simulink model "GolfSwing3D_KineticallyDriven"  (R2025a)
settings: Solver=VariableStepAuto  StartTime=0.0  StopTime=StopTime  MaxStep=0.001  RelTol=1e-3
model workspace: external: MAT-File 3DModelInputs.mat (data not in the file)
undefined symbols (not defined in the file or in its folder): GripStrength, KillswitchFinalValue, KillswitchInitialValue, KillswitchStepTime, LeftLowerArmLength, PlaneTilt, RightLowerArmLength, UpperTorsoLength, X, Y, Z
libraries: nesl_utility x408, sm_lib x139, matrix_library x11, simulink x1
(part 11 of 14)

== matlab function GolfSwing3D_KineticallyDriven/Hip Input Function/Hip Torque Output ==
  data: JointTorqueHipX output; Time input; Killswitch input; HipPositionX input; HipPositionY input; HipPositionZ input; HipVelocityX input; HipVelocityY input; HipVelocityZ input; HipInputXA parameter; HipInputYA parameter; HipInputZA parameter; HipInputXB parameter; HipInputYB parameter; HipInputZB parameter; HipPositionSetpointX parameter; HipPositionSetpointY parameter; GlobalGain parameter; JointTorqueHipY output; JointTorqueHipZ output; HipDampeningX parameter; HipDampeningY parameter; HipDampeningZ parameter; HipConstantX parameter; HipConstantY parameter; HipConstantZ parameter; HipTimeGainX parameter; HipTimeGainY parameter; HipTimeGainZ parameter; HipInputZC parameter; HipInputXC parameter; HipInputYC parameter; HipPositionGainX parameter; HipPositionGainY parameter; HipPositionGainZ parameter; HipPositionSetpointZ parameter; TargetHipPositionX parameter; TargetHipPositionY parameter; TargetHipPositionZ parameter; TargetHipVelocityX parameter; TargetHipVelocityY parameter; TargetHipVelocityZ parameter; HipPCGainX parameter; HipPCGainY parameter; HipPCGainZ parameter; HipVCGainX parameter; HipVCGainY parameter; HipVCGainZ parameter; ModelingMode parameter; ZVCFHipTorqueX parameter; ZVCFHipTorqueY parameter; ZVCFHipTorqueZ parameter; GlobalPCGain parameter; GlobalVCGain parameter; DampeningGlobalGain parameter; TargetImpactTime parameter; HipPositionInputX output; HipPositionInputY output; HipPositionInputZ output; HipVelocityInputX output; HipVelocityInputY output; HipVelocityInputZ output; HipAccelerationInputX output; HipAccelerationInputY output; HipAccelerationInputZ output; HipStartPositionX parameter; HipStartPositionY parameter; HipStartPositionZ parameter; HipStartVelocityX parameter; HipStartVelocityY parameter; HipStartVelocityZ parameter; KinematicMode parameter; HipAoX parameter; HipAoY parameter; HipAoZ parameter; HipAfX parameter; HipAfY parameter; HipAfZ parameter; HipInputXD parameter; HipInputYD parameter; HipInputXE parameter; HipInputXF parameter; HipInputXG parameter; HipInputYE parameter; HipInputYF parameter; HipInputYG parameter; HipInputZD parameter; HipInputZE parameter; HipInputZF parameter; HipInputZG parameter
function [JointTorqueHipX,JointTorqueHipY,JointTorqueHipZ,HipPositionInputX,HipPositionInputY,HipPositionInputZ,HipVelocityInputX,...
    HipVelocityInputY, HipVelocityInputZ,HipAccelerationInputX,HipAccelerationInputY,HipAccelerationInputZ] = fcn(Time,Killswitch, HipPositionX,HipPositionY,HipPositionZ, HipVelocityX,HipVelocityY,...
    HipVelocityZ,...
    HipInputXA,HipInputYA,HipInputZA, HipInputXB,HipInputYB,HipInputZB, HipPositionSetpointX,HipPositionSetpointY,GlobalGain,...
    HipDampeningX, HipDampeningY, HipDampeningZ, HipConstantX, HipConstantY, HipConstantZ, HipTimeGainX, HipTimeGainY, HipTimeGainZ, HipInputZC,...
    HipInputXC, HipInputYC, HipPositionGainX, HipPositionGainY, HipPositionGainZ, HipPositionSetpointZ,...
    TargetHipPositionX, TargetHipPositionY, TargetHipPositionZ, TargetHipVelocityX, TargetHipVelocityY, TargetHipVelocityZ,HipPCGainX, HipPCGainY, HipPCGainZ, HipVCGainX,...
    HipVCGainY, HipVCGainZ,ModelingMode,ZVCFHipTorqueX, ZVCFHipTorqueY, ZVCFHipTorqueZ,GlobalPCGain, GlobalVCGain,DampeningGlobalGain,TargetImpactTime,HipStartPositionX,...
    HipStartPositionY, HipStartPositionZ, HipStartVelocityX, HipStartVelocityY, HipStartVelocityZ,KinematicMode,HipAoX, HipAoY, HipAoZ,HipAfX, HipAfY, HipAfZ,...
    HipInputXD, HipInputYD, HipInputXE, HipInputXF, HipInputXG, HipInputYE, HipInputYF, HipInputYG, HipInputZD, HipInputZE, HipInputZF, HipInputZG)

%Tau=Time/TargetImpactTime;
t=Time;

% %%%%%%%%%%%%%%%%%%%%%%%%%%%%%%%%%%%%%%%%%%%
% % Kinetic Input Selection and Calculation
% %%%%%%%%%%%%%%%%%%%%%%%%%%%%%%%%%%%%%%%%%%%

if ModelingMode==0
    % Values are all set to zero.
    JointTorqueHipX=0;
    JointTorqueHipY=0;
    JointTorqueHipZ=0;
elseif ModelingMode==1
    % Control based strategy. Values are based on difference in value
    % between the current state and desired state.
    % Hip Joint Rotational Deltas
    DeltaHipPositionX=HipPositionX-TargetHipPositionX;
    DeltaHipPositionY=HipPositionY-TargetHipPositionY;
    DeltaHipPositionZ=HipPositionZ-TargetHipPositionZ;
    DeltaHipVelocityX=HipVelocityX-TargetHipVelocityX;
    DeltaHipVelocityY=HipVelocityY-TargetHipVelocityY;
    DeltaHipVelocityZ=HipVelocityZ-TargetHipVelocityZ;
    % Control Based Strategy
    JointTorqueHipX=DeltaHipPositionX*HipPCGainX*GlobalPCGain-DeltaHipVelocityX*HipVCGainX*GlobalVCGain-DampeningGlobalGain*HipDampeningX*HipVelocityX;
    JointTorqueHipY=DeltaHipPositionY*HipPCGainY*GlobalPCGain-DeltaHipVelocityY*HipVCGainY*GlobalVCGain-DampeningGlobalGain*HipDampeningY*HipVelocityY;
    JointTorqueHipZ=DeltaHipPositionZ*HipPCGainZ*GlobalPCGain-DeltaHipVelocityZ*HipVCGainZ*GlobalVCGain-DampeningGlobalGain*HipDampeningZ*HipVelocityZ;
elseif ModelingMode==2
    % Forward Dynamics Based Strategy. Values are computed based on a
    % polynomial and a combination of dampening and position gained
    % factors.
    JointTorqueHipX=Killswitch*GlobalGain*(HipConstantX+HipTimeGainX*Time-HipPositionGainX*(HipPositionX-HipPositionSetpointX)...
    -HipDampeningX*HipVelocityX);
    JointTorqueHipY=Killswitch*GlobalGain*(HipConstantY+HipTimeGainY*Time-HipPositionGainY*(HipPositionY-HipPositionSetpointY)...
    -HipDampeningY*HipVelocityY);
    JointTorqueHipZ=Killswitch*GlobalGain*(HipConstantZ+HipTimeGainZ*Time-HipPositionGainZ*(HipPositionZ-HipPositionSetpointZ)...
    -HipDampeningZ*HipVelocityZ);
elseif ModelingMode==3
    JointTorqueHipX=HexPolyInputFunction(HipInputXA,HipInputXB,HipInputXC,HipInputXD,HipInputXE,HipInputXF,HipInputXG,Time)*Killswitch;
    JointTorqueHipY=HexPolyInputFunction(HipInputYA,HipInputYB,HipInputYC,HipInputYD,HipInputYE,HipInputYF,HipInputYG,Time)*Killswitch;
    JointTorqueHipZ=HexPolyInputFunction(HipInputZA,HipInputZB,HipInputZC,HipInputZD,HipInputZE,HipInputZF,HipInputZG,Time)*Killswitch;
else
    %ZVCF Based Joint Torques. Values are pulled from model workspace and
    %held constant.
    JointTorqueHipX=ZVCFHipTorqueX;
    JointTorqueHipY=ZVCFHipTorqueY;
    JointTorqueHipZ=ZVCFHipTorqueZ;
end

% %%%%%%%%%%%%%%%%%%%%%%%%%%%%%%%%%%%%%%%%%%%
% % Kinematic Input Selection and Calculation
% %%%%%%%%%%%%%%%%%%%%%%%%%%%%%%%%%%%%%%%%%%%

if KinematicMode==0
    % All kinematic values set to zero.
    HipPositionInputX=0;
    HipPositionInputY=0;
    HipPositionInputZ=0;
    HipVelocityInputX=0;
    HipVelocityInputY=0;
    HipVelocityInputZ=0;
    HipAccelerationInputX=0;
    HipAccelerationInputY=0;
    HipAccelerationInputZ=0;
elseif KinematicMode==1
    % 1st Order Acceleration, 2nd Order Velocity, 3rd Order Position Solution
    PTX=TargetHipPositionX;       
    VTX=TargetHipVelocityX;
    PTY=TargetHipPositionY;
    VTY=TargetHipVelocityY;
    PTZ=TargetHipPositionZ;
    VTZ=TargetHipVelocityZ;
    % Define Starting Position and Velocity
    PIX=HipStartPositionX;
    VIX=HipStartVelocityX;
    PIY=HipStartPositionY;
    VIY=HipStartVelocityY;
    PIZ=HipStartPositionZ;
    VIZ=HipStartVelocityZ;
    AX=3*((VTX+VIX)*TargetImpactTime-2*(PTX-PIX))/TargetImpactTime^3;         % Constant in position equation
    BX=-2*((VTX+2*VIX)*TargetImpactTime-3*(PTX-PIX))/TargetImpactTime^2;         % Constant in position equation
    CX=VIX;         % Starting Velocity at Time Zero
    DX=PIX;         % Starting Position at Time Zero
    AY=3*((VTY+VIY)*TargetImpactTime-2*(PTY-PIY))/TargetImpactTime^3;         % Constant in position equation
    BY=-2*((VTY+2*VIY)*TargetImpactTime-3*(PTY-PIY))/TargetImpactTime^2;         % Constant in position equation
    CY=VIY;         % Starting Velocity at Time Zero
    DY=PIY;         % Starting Position at Time Zero
    AZ=3*((VTZ+VIZ)*TargetImpactTime-2*(PTZ-PIZ))/TargetImpactTime^3;         % Constant in position equation
    BZ=-2*((VTZ+2*VIZ)*TargetImpactTime-3*(PTZ-PIZ))/TargetImpactTime^2;         % Constant in position equation
    CZ=VIZ;         % Starting Velocity at Time Zero
    DZ=PIZ;         % Starting Position at Time Zero
    % Equation for position as a function of time
    HipPositionInputX=AX*Time^3/3+BX*Time^2/2+CX*Time+DX;
    HipPositionInputY=AY*Time^3/3+BY*Time^2/2+CY*Time+DY;
    HipPositionInputZ=AZ*Time^3/3+BZ*Time^2/2+CZ*Time+DZ;
    HipVelocityInputX=AX*Time^2+BX*Time+CX;
    HipVelocityInputY=AY*Time^2+BY*Time+CY;
    HipVelocityInputZ=AZ*Time^2+BZ*Time+CZ;
    HipAccelerationInputX=2*AX*Time+BX;
    HipAccelerationInputY=2*AY*Time+BY;
    HipAccelerationInputZ=2*AZ*Time+BZ;
elseif KinematicMode==2
    % 2nd Order Acceleration, 3rd Order Velocity, 4th Order Position Solution
    Tt=TargetImpactTime;
    t=Time;
    PoX=HipStartPositionX;
    PoY=HipStartPositionY;
    PoZ=HipStartPositionZ;
    VoX=HipStartVelocityX;
    VoY=HipStartVelocityY;
    VoZ=HipStartVelocityZ;
    PfX=TargetHipPositionX;
    PfY=TargetHipPositionY;
    PfZ=TargetHipPositionZ;
    VfX=TargetHipVelocityX;
    VfY=TargetHipVelocityY;
    VfZ=TargetHipVelocityZ;
    AoX=HipAoX;
    AoY=HipAoY;
    AoZ=HipAoZ;
    HipPositionInputX=PoX + VoX*t + (AoX*t^2)/2 - (t^3*(4*PoX - 4*PfX + Tt*VfX + 3*Tt*VoX + AoX*Tt^2))/Tt^3 + (t^4*(6*PoX - 6*PfX + 2*Tt*VfX + 4*Tt*VoX + AoX*Tt^2))/(2*Tt^4);
    HipPositionInputY=PoY + VoY*t + (AoY*t^2)/2 - (t^3*(4*PoY - 4*PfY + Tt*VfY + 3*Tt*VoY + AoY*Tt^2))/Tt^3 + (t^4*(6*PoY - 6*PfY + 2*Tt*VfY + 4*Tt*VoY + AoY*Tt^2))/(2*Tt^4);
    HipPositionInputZ=PoZ + VoZ*t + (AoZ*t^2)/2 - (t^3*(4*PoZ - 4*PfZ + Tt*VfZ + 3*Tt*VoZ + AoZ*Tt^2))/Tt^3 + (t^4*(6*PoZ - 6*PfZ + 2*Tt*VfZ + 4*Tt*VoZ + AoZ*Tt^2))/(2*Tt^4);
    HipVelocityInputX=VoX + AoX*t - (3*t^2*(4*PoX - 4*PfX + Tt*VfX + 3*Tt*VoX + AoX*Tt^2))/Tt^3 + (2*t^3*(6*PoX - 6*PfX + 2*Tt*VfX + 4*Tt*VoX + AoX*Tt^2))/Tt^4;
    HipVelocityInputY=VoY + AoY*t - (3*t^2*(4*PoY - 4*PfY + Tt*VfY + 3*Tt*VoY + AoY*Tt^2))/Tt^3 + (2*t^3*(6*PoY - 6*PfY + 2*Tt*VfY + 4*Tt*VoY + AoY*Tt^2))/Tt^4;
    HipVelocityInputZ=VoZ + AoZ*t - (3*t^2*(4*PoZ - 4*PfZ + Tt*VfZ + 3*Tt*VoZ + AoZ*Tt^2))/Tt^3 + (2*t^3*(6*PoZ - 6*PfZ + 2*Tt*VfZ + 4*Tt*VoZ + AoZ*Tt^2))/Tt^4;
    HipAccelerationInputX=AoX + (6*t^2*(6*PoX - 6*PfX + 2*Tt*VfX + 4*Tt*VoX + AoX*Tt^2))/Tt^4 - (6*t*(4*PoX - 4*PfX + Tt*VfX + 3*Tt*VoX + AoX*Tt^2))/Tt^3;
    HipAccelerationInputY=AoY + (6*t^2*(6*PoY - 6*PfY + 2*Tt*VfY + 4*Tt*VoY + AoY*Tt^2))/Tt^4 - (6*t*(4*PoY - 4*PfY + Tt*VfY + 3*Tt*VoY + AoY*Tt^2))/Tt^3;
    HipAccelerationInputZ=AoZ + (6*t^2*(6*PoZ - 6*PfZ + 2*Tt*VfZ + 4*Tt*VoZ + AoZ*Tt^2))/Tt^4 - (6*t*(4*PoZ - 4*PfZ + Tt*VfZ + 3*Tt*VoZ + AoZ*Tt^2))/Tt^3;
else
    % 3rd Order Acceleration, 4th Order Velocity, 5th Order Position Solution
    Tt=TargetImpactTime;
    t=Time;
    PoX=HipStartPositionX;
    PoY=HipStartPositionY;
    PoZ=HipStartPositionZ;
    VoX=HipStartVelocityX;
    VoY=HipStartVelocityY;
    VoZ=HipStartVelocityZ;
    PfX=TargetHipPositionX;
    PfY=TargetHipPositionY;
    PfZ=TargetHipPositionZ;
    VfX=TargetHipVelocityX;
    VfY=TargetHipVelocityY;
    VfZ=TargetHipVelocityZ;
    AoX=HipAoX;
    AoY=HipAoY;
    AoZ=HipAoZ;
    AfX=HipAfX;
    AfY=HipAfY;
    AfZ=HipAfZ;
    HipPositionInputX=PoX+VoX*t+(AoX*t^2)/2-(t^5*(12*PoX-12*PfX+6*Tt*VfX+6*Tt*VoX-AfX*Tt^2+AoX*Tt^2))/(2*Tt^5)-(t^3*(20*PoX-20*PfX+8*Tt*VfX+12*Tt*VoX-AfX*Tt^2+3*AoX*Tt^2))/(2*Tt^3)+(t^4*(30*PoX-30*PfX+14*Tt*VfX+16*Tt*VoX-2*AfX*Tt^2+3*AoX*Tt^2))/(2*Tt^4);
    HipPositionInputY=PoY+VoY*t+(AoY*t^2)/2-(t^5*(12*PoY-12*PfY+6*Tt*VfY+6*Tt*VoY-AfY*Tt^2+AoY*Tt^2))/(2*Tt^5)-(t^3*(20*PoY-20*PfY+8*Tt*VfY+12*Tt*VoY-AfY*Tt^2+3*AoY*Tt^2))/(2*Tt^3)+(t^4*(30*PoY-30*PfY+14*Tt*VfY+16*Tt*VoY-2*AfY*Tt^2+3*AoY*Tt^2))/(2*Tt^4);  
    HipPositionInputZ=PoZ+VoZ*t+(AoZ*t^2)/2-(t^5*(12*PoZ-12*PfZ+6*Tt*VfZ+6*Tt*VoZ-AfZ*Tt^2+AoZ*Tt^2))/(2*Tt^5)-(t^3*(20*PoZ-20*PfZ+8*Tt*VfZ+12*Tt*VoZ-AfZ*Tt^2+3*AoZ*Tt^2))/(2*Tt^3)+(t^4*(30*PoZ-30*PfZ+14*Tt*VfZ+16*Tt*VoZ-2*AfZ*Tt^2+3*AoZ*Tt^2))/(2*Tt^4);
    HipVelocityInputX=VoX+AoX*t-(5*t^4*(12*PoX-12*PfX+6*Tt*VfX+6*Tt*VoX-AfX*Tt^2+AoX*Tt^2))/(2*Tt^5)-(3*t^2*(20*PoX-20*PfX+8*Tt*VfX+12*Tt*VoX-AfX*Tt^2+3*AoX*Tt^2))/(2*Tt^3)+(2*t^3*(30*PoX-30*PfX+14*Tt*VfX+16*Tt*VoX-2*AfX*Tt^2+3*AoX*Tt^2))/Tt^4;
    HipVelocityInputY=VoY+AoY*t-(5*t^4*(12*PoY-12*PfY+6*Tt*VfY+6*Tt*VoY-AfY*Tt^2+AoY*Tt^2))/(2*Tt^5)-(3*t^2*(20*PoY-20*PfY+8*Tt*VfY+12*Tt*VoY-AfY*Tt^2+3*AoY*Tt^2))/(2*Tt^3)+(2*t^3*(30*PoY-30*PfY+14*Tt*VfY+16*Tt*VoY-2*AfY*Tt^2+3*AoY*Tt^2))/Tt^4;
    HipVelocityInputZ=VoZ+AoZ*t-(5*t^4*(12*PoZ-12*PfZ+6*Tt*VfZ+6*Tt*VoZ-AfZ*Tt^2+AoZ*Tt^2))/(2*Tt^5)-(3*t^2*(20*PoZ-20*PfZ+8*Tt*VfZ+12*Tt*VoZ-AfZ*Tt^2+3*AoZ*Tt^2))/(2*Tt^3)+(2*t^3*(30*PoZ-30*PfZ+14*Tt*VfZ+16*Tt*VoZ-2*AfZ*Tt^2+3*AoZ*Tt^2))/Tt^4;
    HipAccelerationInputX=AoX-(3*t*(20*PoX-20*PfX+8*Tt*VfX+12*Tt*VoX-AfX*Tt^2+3*AoX*Tt^2))/Tt^3-(10*t^3*(12*PoX-12*PfX+6*Tt*VfX+6*Tt*VoX-AfX*Tt^2+AoX*Tt^2))/Tt^5+(6*t^2*(30*PoX-30*PfX+14*Tt*VfX+16*Tt*VoX-2*AfX*Tt^2+3*AoX*Tt^2))/Tt^4;
    HipAccelerationInputY=AoY-(3*t*(20*PoY-20*PfY+8*Tt*VfY+12*Tt*VoY-AfY*Tt^2+3*AoY*Tt^2))/Tt^3-(10*t^3*(12*PoY-12*PfY+6*Tt*VfY+6*Tt*VoY-AfY*Tt^2+AoY*Tt^2))/Tt^5+(6*t^2*(30*PoY-30*PfY+14*Tt*VfY+16*Tt*VoY-2*AfY*Tt^2+3*AoY*Tt^2))/Tt^4;
    HipAccelerationInputZ=AoZ-(3*t*(20*PoZ-20*PfZ+8*Tt*VfZ+12*Tt*VoZ-AfZ*Tt^2+3*AoZ*Tt^2))/Tt^3-(10*t^3*(12*PoZ-12*PfZ+6*Tt*VfZ+6*Tt*VoZ-AfZ*Tt^2+AoZ*Tt^2))/Tt^5+(6*t^2*(30*PoZ-30*PfZ+14*Tt*VfZ+16*Tt*VoZ-2*AfZ*Tt^2+3*AoZ*Tt^2))/Tt^4;
end

% Calculate Higher Order Derivatives of the Position Outputs
HipJerkX=gradient(HipAccelerationInputX,t);
HipJerkY=gradient(HipAccelerationInputY,t);
HipJerkZ=gradient(HipAccelerationInputZ,t);
HipSnapX=gradient(HipJerkX,t);
HIpSnapY=gradient(HipJerkY,t);
HipSnapZ=gradient(HipJerkZ,t);
HipCrackleX=gradient(HipSnapX,t);
HipCrackleY=gradient(HIpSnapY,t);
HipCrackleZ=gradient(HipSnapZ,t);
HipPopX=gradient(HipCrackleX,t);
HipPopY=gradient(HipCrackleY,t);
HipPopZ=gradient(HipCrackleZ,t);

== matlab function GolfSwing3D_KineticallyDriven/Club Calculations/Subsystem/Total Wrist Forces and Torques Local ==
  data: LHTL input; RHTL input; LHTG input; RHTG input; LHFL input; RHFL input; LHFG input; RHFG input; HandPathVector input; MidpointVelocity input; TotalHandTorqueLocal output; TotalHandTorqueGlobal output; ClubTorqueMagnitude output; TotalHandForceLocal output; TotalHandForceGlobal output; ClubForceMagnitude output; HandForceYankLocal output; ForceAlongHandPath output; LinearPoweronClub output; LHAV input; RHAV input; LHonClubAngularPower output; RHonClubAngularPower output; LHMOF input; RHMOF input; SumofMomentsLHonClub output; SumofMomentsRHonClub output; LHVelocity input; RHVelocity input; LHandPathVector input; RHandPathVector input; LHonClubLinearPower output; RHonClubLinearPower output; LHForceAlongHandPath output; RHForceAlongHandPath output
function [TotalHandTorqueLocal,TotalHandTorqueGlobal,ClubTorqueMagnitude,TotalHandForceLocal,TotalHandForceGlobal,...
    ClubForceMagnitude,HandForceYankLocal,ForceAlongHandPath,LinearPoweronClub,...
    LHonClubAngularPower,RHonClubAngularPower,SumofMomentsLHonClub,SumofMomentsRHonClub,...
    LHonClubLinearPower,RHonClubLinearPower,LHForceAlongHandPath,RHForceAlongHandPath] = ...
    fcn(LHTL,RHTL,LHTG,RHTG,LHFL,RHFL,LHFG,RHFG,HandPathVector,MidpointVelocity,LHAV,RHAV,LHMOF,RHMOF,...
    LHVelocity,RHVelocity,LHandPathVector,RHandPathVector)

% Local Torques
TotalHandTorqueLocal = LHTL+RHTL;
ClubTorqueMagnitude=norm(TotalHandTorqueLocal);

% Local Forces
TotalHandForceLocal = LHFL+RHFL;
ClubForceMagnitude=norm(TotalHandForceLocal);
HandForceYankLocal=diff(TotalHandForceLocal);

% Global Torques
TotalHandTorqueGlobal=LHTG+RHTG;

% Global Forces
TotalHandForceGlobal=LHFG+RHFG;

% Force Along Hand Path
ForceAlongHandPath=dot(TotalHandForceGlobal,HandPathVector);
LHForceAlongHandPath=dot(LHFG,LHandPathVector);
RHForceAlongHandPath=dot(RHFG,RHandPathVector);

% Linear Power Applied to Club
LinearPoweronClub=dot(TotalHandForceGlobal,MidpointVelocity);
LHonClubLinearPower=dot(LHFG,LHVelocity);
RHonClubLinearPower=dot(RHFG,RHVelocity);

% Angular Power
LHonClubAngularPower=dot(LHTG,LHAV);
RHonClubAngularPower=dot(RHTG,RHAV);

% Sum of Moments
SumofMomentsLHonClub=LHMOF+LHTG;
SumofMomentsRHonClub=RHMOF+RHTG;

== matlab function GolfSwing3D_KineticallyDriven/Torso Input Function/Torso Input Torque ==
  data: Time input; Killswitch input; JointTorqueTorso output; TorsoInputB parameter; TorsoPositionSetpoint parameter; GlobalGain parameter; TorsoDampening parameter; ModelingMode parameter; GlobalPCGain parameter; GlobalVCGain parameter; DampeningGlobalGain parameter; TargetImpactTime parameter; KinematicMode parameter; TorsoAo parameter; TorsoStartPosition parameter; TorsoStartVelocity parameter; ZVCFTorsoTorque parameter; TorsoPCGain parameter; TorsoVCGain parameter; TargetTorsoVelocity parameter; TargetTorsoPosition parameter; TorsoPositionGain parameter; TorsoPositionInput output; TorsoVelocityInput output; TorsoAccelerationInput output; TorsoInputC parameter; TorsoTimeGain parameter; TorsoConstant parameter; TorsoPosition input; TorsoVelocity input; TorsoInputA parameter; TorsoAf parameter; TorsoInputD parameter; TorsoInputE parameter; TorsoInputF parameter; TorsoInputG parameter
function [JointTorqueTorso,TorsoPositionInput,TorsoVelocityInput,...
    TorsoAccelerationInput]  = fcn(Time,Killswitch,...
    TorsoInputB,TorsoPositionSetpoint,GlobalGain,...
    TorsoDampening, ModelingMode,GlobalPCGain, GlobalVCGain,...
    DampeningGlobalGain,TargetImpactTime,KinematicMode, TorsoAo,TorsoStartPosition,...
    TorsoStartVelocity,ZVCFTorsoTorque,TorsoPCGain,TorsoVCGain,...
    TargetTorsoVelocity,TargetTorsoPosition, ...
    TorsoPositionGain,TorsoInputC,...
    TorsoTimeGain, TorsoConstant,TorsoPosition,TorsoVelocity, TorsoInputA,TorsoAf,TorsoInputD, TorsoInputE, TorsoInputF, TorsoInputG)

%Tau=Time/TargetImpactTime;
t=Time;

% %%%%%%%%%%%%%%%%%%%%%%%%%%%%%%%%%%%%%%%%%%%
% % Kinetic Input Selection and Calculation
% %%%%%%%%%%%%%%%%%%%%%%%%%%%%%%%%%%%%%%%%%%%

if ModelingMode==0
    % Values are all set to zero.
    JointTorqueTorso=0;
elseif ModelingMode==1
    % Control based strategy. Values are based on difference in value
    % between the current state and desired state.
    % Torso Joint Rotational Deltas
    DeltaTorsoPosition=TorsoPosition-TargetTorsoPosition;
    DeltaTorsoVelocity=TorsoVelocity-TargetTorsoVelocity;
    % Control Based Strategy
    JointTorqueTorso=DeltaTorsoPosition*TorsoPCGain*GlobalPCGain-DeltaTorsoVelocity*TorsoVCGain*GlobalVCGain-DampeningGlobalGain*TorsoDampening*TorsoVelocity;
elseif ModelingMode==2
    % Forward Dynamics Based Strategy. Values are computed based on a
    % polynomial and a combination of dampening and position gained
    % factors.
    JointTorqueTorso=Killswitch*GlobalGain*(TorsoConstant+TorsoTimeGain*Time-TorsoPositionGain*(TorsoPosition-TorsoPositionSetpoint)...
    -TorsoDampening*TorsoVelocity);
elseif ModelingMode==3
    JointTorqueTorso=HexPolyInputFunction(TorsoInputA,TorsoInputB,TorsoInputC,TorsoInputD,TorsoInputE,TorsoInputF,TorsoInputG,Time)*Killswitch;
else
    %ZVCF Based Joint Torques. Values are pulled from model workspace and
    %held constant.
    JointTorqueTorso=ZVCFTorsoTorque;
end

% %%%%%%%%%%%%%%%%%%%%%%%%%%%%%%%%%%%%%%%%%%%
% % Kinematic Input Selection and Calculation
% %%%%%%%%%%%%%%%%%%%%%%%%%%%%%%%%%%%%%%%%%%%

if KinematicMode==0
    % All kinematic values set to zero.
    TorsoPositionInput=0;
    TorsoPositionInputY=0;
    TorsoVelocityInput=0;
    TorsoVelocityInputY=0;
    TorsoAccelerationInput=0;
    TorsoAccelerationInputY=0;
elseif KinematicMode==1
    % 1st Order Acceleration, 2nd Order Velocity, 3rd Order Position Solution
    PTX=TargetTorsoPosition;       
    VTX=TargetTorsoVelocity;
    % Define Starting Position and Velocity
    PIX=TorsoStartPosition;
    VIX=TorsoStartVelocity;
    AX=3*((VTX+VIX)*TargetImpactTime-2*(PTX-PIX))/TargetImpactTime^3;         % Constant in position equation
    BX=-2*((VTX+2*VIX)*TargetImpactTime-3*(PTX-PIX))/TargetImpactTime^2;         % Constant in position equation
    CX=VIX;         % Starting Velocity at Time Zero
    DX=PIX;         % Starting Position at Time Zero
    % Equation for position as a function of time
    TorsoPositionInput=AX*Time^3/3+BX*Time^2/2+CX*Time+DX;
    TorsoVelocityInput=AX*Time^2+BX*Time+CX;
    TorsoAccelerationInput=2*AX*Time+BX;
elseif KinematicMode==2
    % 2nd Order Acceleration, 3rd Order Velocity, 4th Order Position Solution
    Tt=TargetImpactTime;
    t=Time;
    PoX=TorsoStartPosition;
    VoX=TorsoStartVelocity;
    PfX=TargetTorsoPosition;
    VfX=TargetTorsoVelocity;
    AoX=TorsoAo;
    TorsoPositionInput=PoX + VoX*t + (AoX*t^2)/2 - (t^3*(4*PoX - 4*PfX + Tt*VfX + 3*Tt*VoX + AoX*Tt^2))/Tt^3 + (t^4*(6*PoX - 6*PfX + 2*Tt*VfX + 4*Tt*VoX + AoX*Tt^2))/(2*Tt^4);
    TorsoVelocityInput=VoX + AoX*t - (3*t^2*(4*PoX - 4*PfX + Tt*VfX + 3*Tt*VoX + AoX*Tt^2))/Tt^3 + (2*t^3*(6*PoX - 6*PfX + 2*Tt*VfX + 4*Tt*VoX + AoX*Tt^2))/Tt^4;
    TorsoAccelerationInput=AoX + (6*t^2*(6*PoX - 6*PfX + 2*Tt*VfX + 4*Tt*VoX + AoX*Tt^2))/Tt^4 - (6*t*(4*PoX - 4*PfX + Tt*VfX + 3*Tt*VoX + AoX*Tt^2))/Tt^3;
else
    % 3rd Order Acceleration, 4th Order Velocity, 5th Order Position Solution
    Tt=TargetImpactTime;
    t=Time;
    PoX=TorsoStartPosition;
    VoX=TorsoStartVelocity;
    PfX=TargetTorsoPosition;
    VfX=TargetTorsoVelocity;
    AoX=TorsoAo;
    AfX=TorsoAf;
    TorsoPositionInput=PoX+VoX*t+(AoX*t^2)/2-(t^5*(12*PoX-12*PfX+6*Tt*VfX+6*Tt*VoX-AfX*Tt^2+AoX*Tt^2))/(2*Tt^5)-(t^3*(20*PoX-20*PfX+8*Tt*VfX+12*Tt*VoX-AfX*Tt^2+3*AoX*Tt^2))/(2*Tt^3)+(t^4*(30*PoX-30*PfX+14*Tt*VfX+16*Tt*VoX-2*AfX*Tt^2+3*AoX*Tt^2))/(2*Tt^4);
    TorsoVelocityInput=VoX+AoX*t-(5*t^4*(12*PoX-12*PfX+6*Tt*VfX+6*Tt*VoX-AfX*Tt^2+AoX*Tt^2))/(2*Tt^5)-(3*t^2*(20*PoX-20*PfX+8*Tt*VfX+12*Tt*VoX-AfX*Tt^2+3*AoX*Tt^2))/(2*Tt^3)+(2*t^3*(30*PoX-30*PfX+14*Tt*VfX+16*Tt*VoX-2*AfX*Tt^2+3*AoX*Tt^2))/Tt^4;
    TorsoAccelerationInput=AoX-(3*t*(20*PoX-20*PfX+8*Tt*VfX+12*Tt*VoX-AfX*Tt^2+3*AoX*Tt^2))/Tt^3-(10*t^3*(12*PoX-12*PfX+6*Tt*VfX+6*Tt*VoX-AfX*Tt^2+AoX*Tt^2))/Tt^5+(6*t^2*(30*PoX-30*PfX+14*Tt*VfX+16*Tt*VoX-2*AfX*Tt^2+3*AoX*Tt^2))/Tt^4;
end


% Calculate Higher Order Derivatives of the Position Outputs
TorsoJerk=gradient(TorsoAccelerationInput,t);
TorsoSnap=gradient(TorsoJerk,t);
TorsoCrackle=gradient(TorsoSnap,t);
TorsoPop=gradient(TorsoCrackle,t);

== matlab function GolfSwing3D_KineticallyDriven/LScap Input Function/LScap Torque ==
  data: Time input; Killswitch input; JointTorqueLScapX output; LScapInputXA parameter; LScapInputYA parameter; LScapInputXB parameter; LScapInputYB parameter; LScapPositionSetpointX parameter; GlobalGain parameter; LScapConstantX parameter; JointTorqueLScapY output; LScapPositionInputX output; LScapPositionInputY output; LScapVelocityInputX output; LScapConstantY parameter; LScapTimeGainX parameter; LScapTimeGainY parameter; LScapInputXC parameter; LScapInputYC parameter; LScapPositionGainX parameter; LScapPositionGainY parameter; TargetLScapPositionX parameter; ModelingMode parameter; GlobalPCGain parameter; GlobalVCGain parameter; DampeningGlobalGain parameter; TargetImpactTime parameter; LScapAoX parameter; LScapAoY parameter; KinematicMode parameter; LScapDampeningX parameter; LScapDampeningY parameter; LScapPositionSetpointY parameter; LScapStartPositionX parameter; LScapStartPositionY parameter; LScapStartVelocityX parameter; LScapStartVelocityY parameter; LScapVCGainX parameter; LScapVCGainY parameter; LScapVelocityInputY output; LScapAccelerationInputX output; LScapAccelerationInputY output; LScapPCGainX parameter; LScapPCGainY parameter; LScapPositionX input; LScapPositionY input; LScapVelocityX input; LScapVelocityY input; ZVCFLScapTorqueX parameter; ZVCFLScapTorqueY parameter; TargetLScapPositionY parameter; TargetLScapVelocityX parameter; TargetLScapVelocityY parameter; LScapAfX parameter; LScapAfY parameter; LScapInputXD parameter; LScapInputXE parameter; LScapInputXF parameter; LScapInputXG parameter; LScapInputYD parameter; LScapInputYE parameter; LScapInputYF parameter; LScapInputYG parameter
function [JointTorqueLScapX,JointTorqueLScapY,LScapPositionInputX, LScapPositionInputY, LScapVelocityInputX,LScapVelocityInputY,LScapAccelerationInputX,LScapAccelerationInputY] = fcn(Time,Killswitch, LScapInputXA,LScapInputYA, LScapInputXB,LScapInputYB, LScapPositionSetpointX,GlobalGain,...
    LScapConstantX, LScapConstantY, LScapTimeGainX, LScapTimeGainY,...
    LScapInputXC, LScapInputYC, LScapPositionGainX, LScapPositionGainY,...
    TargetLScapPositionX, ModelingMode,GlobalPCGain, GlobalVCGain,DampeningGlobalGain,TargetImpactTime,LScapAoX, LScapAoY, KinematicMode, LScapDampeningX, LScapDampeningY, LScapPositionSetpointY, LScapStartPositionX,...
    LScapStartPositionY, LScapStartVelocityX, LScapStartVelocityY, LScapVCGainX,...
    LScapVCGainY, LScapPCGainX, LScapPCGainY, LScapPositionX, LScapPositionY, LScapVelocityX,...
    LScapVelocityY, ZVCFLScapTorqueX, ZVCFLScapTorqueY, TargetLScapPositionY, TargetLScapVelocityX,...
    TargetLScapVelocityY,LScapAfX, LScapAfY,LScapInputXD, LScapInputXE, LScapInputXF, LScapInputXG,...
LScapInputYD, LScapInputYE, LScapInputYF, LScapInputYG)

%Tau=Time/TargetImpactTime;
t=Time;

% %%%%%%%%%%%%%%%%%%%%%%%%%%%%%%%%%%%%%%%%%%%
% % Kinetic Input Selection and Calculation
% %%%%%%%%%%%%%%%%%%%%%%%%%%%%%%%%%%%%%%%%%%%

if ModelingMode==0
    % Values are all set to zero.
    JointTorqueLScapX=0;
    JointTorqueLScapY=0;
elseif ModelingMode==1
    % Control based strategy. Values are based on difference in value
    % between the current state and desired state.
    % LScap Joint Rotational Deltas
    DeltaLScapPositionX=LScapPositionX-TargetLScapPositionX;
    DeltaLScapPositionY=LScapPositionY-TargetLScapPositionY;
    DeltaLScapVelocityX=LScapVelocityX-TargetLScapVelocityX;
    DeltaLScapVelocityY=LScapVelocityY-TargetLScapVelocityY;
    % Control Based Strategy
    JointTorqueLScapX=DeltaLScapPositionX*LScapPCGainX*GlobalPCGain-DeltaLScapVelocityX*LScapVCGainX*GlobalVCGain-DampeningGlobalGain*LScapDampeningX*LScapVelocityX;
    JointTorqueLScapY=DeltaLScapPositionY*LScapPCGainY*GlobalPCGain-DeltaLScapVelocityY*LScapVCGainY*GlobalVCGain-DampeningGlobalGain*LScapDampeningY*LScapVelocityY;
elseif ModelingMode==2
    % Forward Dynamics Based Strategy. Values are computed based on a
    % polynomial and a combination of dampening and position gained
    % factors.
    JointTorqueLScapX=Killswitch*GlobalGain*(LScapConstantX+LScapTimeGainX*Time-LScapPositionGainX*(LScapPositionX-LScapPositionSetpointX)...
    -LScapDampeningX*LScapVelocityX);
    JointTorqueLScapY=Killswitch*GlobalGain*(LScapConstantY+LScapTimeGainY*Time-LScapPositionGainY*(LScapPositionY-LScapPositionSetpointY)...
    -LScapDampeningY*LScapVelocityY);
elseif ModelingMode==3
    JointTorqueLScapX=HexPolyInputFunction(LScapInputXA,LScapInputXB,LScapInputXC,LScapInputXD,LScapInputXE,LScapInputXF,LScapInputXG,Time)*Killswitch;
    JointTorqueLScapY=HexPolyInputFunction(LScapInputYA,LScapInputYB,LScapInputYC,LScapInputYD,LScapInputYE,LScapInputYF,LScapInputYG,Time)*Killswitch; 
else
    %ZVCF Based Joint Torques. Values are pulled from model workspace and
    %held constant.
    JointTorqueLScapX=ZVCFLScapTorqueX;
    JointTorqueLScapY=ZVCFLScapTorqueY;
end

% %%%%%%%%%%%%%%%%%%%%%%%%%%%%%%%%%%%%%%%%%%%
% % Kinematic Input Selection and Calculation
% %%%%%%%%%%%%%%%%%%%%%%%%%%%%%%%%%%%%%%%%%%%

if KinematicMode==0
    % All kinematic values set to zero.
    LScapPositionInputX=0;
    LScapPositionInputY=0;
    LScapVelocityInputX=0;
    LScapVelocityInputY=0;
    LScapAccelerationInputX=0;
    LScapAccelerationInputY=0;
elseif KinematicMode==1
    % 1st Order Acceleration, 2nd Order Velocity, 3rd Order Position Solution
    PTX=TargetLScapPositionX;       
    VTX=TargetLScapVelocityX;
    PTY=TargetLScapPositionY;
    VTY=TargetLScapVelocityY;
    % Define Starting Position and Velocity
    PIX=LScapStartPositionX;
    VIX=LScapStartVelocityX;
    PIY=LScapStartPositionY;
    VIY=LScapStartVelocityY;
    AX=3*((VTX+VIX)*TargetImpactTime-2*(PTX-PIX))/TargetImpactTime^3;         % Constant in position equation
    BX=-2*((VTX+2*VIX)*TargetImpactTime-3*(PTX-PIX))/TargetImpactTime^2;         % Constant in position equation
    CX=VIX;         % Starting Velocity at Time Zero
    DX=PIX;         % Starting Position at Time Zero
    AY=3*((VTY+VIY)*TargetImpactTime-2*(PTY-PIY))/TargetImpactTime^3;         % Constant in position equation
    BY=-2*((VTY+2*VIY)*TargetImpactTime-3*(PTY-PIY))/TargetImpactTime^2;         % Constant in position equation
    CY=VIY;         % Starting Velocity at Time Zero
    DY=PIY;         % Starting Position at Time Zero
    % Equation for position as a function of time
    LScapPositionInputX=AX*Time^3/3+BX*Time^2/2+CX*Time+DX;
    LScapPositionInputY=AY*Time^3/3+BY*Time^2/2+CY*Time+DY;
    LScapVelocityInputX=AX*Time^2+BX*Time+CX;
    LScapVelocityInputY=AY*Time^2+BY*Time+CY;
    LScapAccelerationInputX=2*AX*Time+BX;
    LScapAccelerationInputY=2*AY*Time+BY;
elseif KinematicMode==2
    % 2nd Order Acceleration, 3rd Order Velocity, 4th Order Position Solution
    Tt=TargetImpactTime;
    t=Time;
    PoX=LScapStartPositionX;
    PoY=LScapStartPositionY;
    VoX=LScapStartVelocityX;
    VoY=LScapStartVelocityY;
    PfX=TargetLScapPositionX;
    PfY=TargetLScapPositionY;
    VfX=TargetLScapVelocityX;
    VfY=TargetLScapVelocityY;
    AoX=LScapAoX;
    AoY=LScapAoY;
    LScapPositionInputX=PoX + VoX*t + (AoX*t^2)/2 - (t^3*(4*PoX - 4*PfX + Tt*VfX + 3*Tt*VoX + AoX*Tt^2))/Tt^3 + (t^4*(6*PoX - 6*PfX + 2*Tt*VfX + 4*Tt*VoX + AoX*Tt^2))/(2*Tt^4);
    LScapPositionInputY=PoY + VoY*t + (AoY*t^2)/2 - (t^3*(4*PoY - 4*PfY + Tt*VfY + 3*Tt*VoY + AoY*Tt^2))/Tt^3 + (t^4*(6*PoY - 6*PfY + 2*Tt*VfY + 4*Tt*VoY + AoY*Tt^2))/(2*Tt^4);
    LScapVelocityInputX=VoX + AoX*t - (3*t^2*(4*PoX - 4*PfX + Tt*VfX + 3*Tt*VoX + AoX*Tt^2))/Tt^3 + (2*t^3*(6*PoX - 6*PfX + 2*Tt*VfX + 4*Tt*VoX + AoX*Tt^2))/Tt^4;
    LScapVelocityInputY=VoY + AoY*t - (3*t^2*(4*PoY - 4*PfY + Tt*VfY + 3*Tt*VoY + AoY*Tt^2))/Tt^3 + (2*t^3*(6*PoY - 6*PfY + 2*Tt*VfY + 4*Tt*VoY + AoY*Tt^2))/Tt^4;
    LScapAccelerationInputX=AoX + (6*t^2*(6*PoX - 6*PfX + 2*Tt*VfX + 4*Tt*VoX + AoX*Tt^2))/Tt^4 - (6*t*(4*PoX - 4*PfX + Tt*VfX + 3*Tt*VoX + AoX*Tt^2))/Tt^3;
    LScapAccelerationInputY=AoY + (6*t^2*(6*PoY - 6*PfY + 2*Tt*VfY + 4*Tt*VoY + AoY*Tt^2))/Tt^4 - (6*t*(4*PoY - 4*PfY + Tt*VfY + 3*Tt*VoY + AoY*Tt^2))/Tt^3;
else
    % 3rd Order Acceleration, 4th Order Velocity, 5th Order Position Solution
    Tt=TargetImpactTime;
    t=Time;
    PoX=LScapStartPositionX;
    PoY=LScapStartPositionY;
    VoX=LScapStartVelocityX;
    VoY=LScapStartVelocityY;
    PfX=TargetLScapPositionX;
    PfY=TargetLScapPositionY;
    VfX=TargetLScapVelocityX;
    VfY=TargetLScapVelocityY;
    AoX=LScapAoX;
    AoY=LScapAoY;
    AfX=LScapAfX;
    AfY=LScapAfY;
    LScapPositionInputX=PoX+VoX*t+(AoX*t^2)/2-(t^5*(12*PoX-12*PfX+6*Tt*VfX+6*Tt*VoX-AfX*Tt^2+AoX*Tt^2))/(2*Tt^5)-(t^3*(20*PoX-20*PfX+8*Tt*VfX+12*Tt*VoX-AfX*Tt^2+3*AoX*Tt^2))/(2*Tt^3)+(t^4*(30*PoX-30*PfX+14*Tt*VfX+16*Tt*VoX-2*AfX*Tt^2+3*AoX*Tt^2))/(2*Tt^4);
    LScapPositionInputY=PoY+VoY*t+(AoY*t^2)/2-(t^5*(12*PoY-12*PfY+6*Tt*VfY+6*Tt*VoY-AfY*Tt^2+AoY*Tt^2))/(2*Tt^5)-(t^3*(20*PoY-20*PfY+8*Tt*VfY+12*Tt*VoY-AfY*Tt^2+3*AoY*Tt^2))/(2*Tt^3)+(t^4*(30*PoY-30*PfY+14*Tt*VfY+16*Tt*VoY-2*AfY*Tt^2+3*AoY*Tt^2))/(2*Tt^4);  
    LScapVelocityInputX=VoX+AoX*t-(5*t^4*(12*PoX-12*PfX+6*Tt*VfX+6*Tt*VoX-AfX*Tt^2+AoX*Tt^2))/(2*Tt^5)-(3*t^2*(20*PoX-20*PfX+8*Tt*VfX+12*Tt*VoX-AfX*Tt^2+3*AoX*Tt^2))/(2*Tt^3)+(2*t^3*(30*PoX-30*PfX+14*Tt*VfX+16*Tt*VoX-2*AfX*Tt^2+3*AoX*Tt^2))/Tt^4;
    LScapVelocityInputY=VoY+AoY*t-(5*t^4*(12*PoY-12*PfY+6*Tt*VfY+6*Tt*VoY-AfY*Tt^2+AoY*Tt^2))/(2*Tt^5)-(3*t^2*(20*PoY-20*PfY+8*Tt*VfY+12*Tt*VoY-AfY*Tt^2+3*AoY*Tt^2))/(2*Tt^3)+(2*t^3*(30*PoY-30*PfY+14*Tt*VfY+16*Tt*VoY-2*AfY*Tt^2+3*AoY*Tt^2))/Tt^4;
    LScapAccelerationInputX=AoX-(3*t*(20*PoX-20*PfX+8*Tt*VfX+12*Tt*VoX-AfX*Tt^2+3*AoX*Tt^2))/Tt^3-(10*t^3*(12*PoX-12*PfX+6*Tt*VfX+6*Tt*VoX-AfX*Tt^2+AoX*Tt^2))/Tt^5+(6*t^2*(30*PoX-30*PfX+14*Tt*VfX+16*Tt*VoX-2*AfX*Tt^2+3*AoX*Tt^2))/Tt^4;
    LScapAccelerationInputY=AoY-(3*t*(20*PoY-20*PfY+8*Tt*VfY+12*Tt*VoY-AfY*Tt^2+3*AoY*Tt^2))/Tt^3-(10*t^3*(12*PoY-12*PfY+6*Tt*VfY+6*Tt*VoY-AfY*Tt^2+AoY*Tt^2))/Tt^5+(6*t^2*(30*PoY-30*PfY+14*Tt*VfY+16*Tt*VoY-2*AfY*Tt^2+3*AoY*Tt^2))/Tt^4;
end

% Calculate Higher Order Derivatives of the Position Outputs
LScapJerkX=gradient(LScapAccelerationInputX,t);
LScapJerkY=gradient(LScapAccelerationInputY,t);
LScapSnapX=gradient(LScapJerkX,t);
LScapSnapY=gradient(LScapJerkY,t);
LScapCrackleX=gradient(LScapSnapX,t);
LScapCrackleY=gradient(LScapSnapY,t);
LScapPopX=gradient(LScapCrackleX,t);
LScapPopY=gradient(LScapCrackleY,t);

== matlab function GolfSwing3D_KineticallyDriven/RScap Input Function/RScap Torque ==
  data: Time input; Killswitch input; JointTorqueRScapX output; RScapInputXA parameter; RScapInputYA parameter; RScapInputXB parameter; RScapInputYB parameter; RScapPositionSetpointX parameter; GlobalGain parameter; RScapConstantX parameter; JointTorqueRScapY output; RScapConstantY parameter; RScapTimeGainX parameter; RScapTimeGainY parameter; RScapInputXC parameter; RScapInputYC parameter; RScapPositionGainX parameter; RScapPositionGainY parameter; TargetRScapPositionX parameter; ModelingMode parameter; GlobalPCGain parameter; GlobalVCGain parameter; DampeningGlobalGain parameter; TargetImpactTime parameter; KinematicMode parameter; RScapPositionSetpointY parameter; RScapStartPositionX parameter; RScapStartPositionY parameter; RScapVCGainX parameter; RScapVCGainY parameter; RScapPCGainX parameter; RScapPCGainY parameter; RScapPositionInputX output; RScapPositionInputY output; RScapVelocityInputX output; RScapVelocityInputY output; RScapAccelerationInputX output; RScapAccelerationInputY output; ZVCFRScapTorqueX parameter; ZVCFRScapTorqueY parameter; TargetRScapPositionY parameter; TargetRScapVelocityX parameter; TargetRScapVelocityY parameter; RScapAoX parameter; RScapAoY parameter; RScapDampeningX parameter; RScapDampeningY parameter; RScapPositionX input; RScapPositionY input; RScapVelocityX input; RScapVelocityY input; RScapStartVelocityX parameter; RScapStartVelocityY parameter; RScapAfX parameter; RScapAfY parameter; RScapInputXD parameter; RScapInputXE parameter; RScapInputXF parameter; RScapInputXG parameter; RScapInputYD parameter; RScapInputYE parameter; RScapInputYF parameter; RScapInputYG parameter
function [JointTorqueRScapX,JointTorqueRScapY,RScapPositionInputX,...
    RScapPositionInputY, RScapVelocityInputX,RScapVelocityInputY,...
    RScapAccelerationInputX,RScapAccelerationInputY] = fcn(Time,Killswitch,...
    RScapInputXA,RScapInputYA, RScapInputXB,RScapInputYB, RScapPositionSetpointX,GlobalGain,...
    RScapConstantX, RScapConstantY, RScapTimeGainX, RScapTimeGainY,...
    RScapInputXC, RScapInputYC, RScapPositionGainX, RScapPositionGainY,...
    TargetRScapPositionX, ModelingMode,GlobalPCGain, GlobalVCGain,DampeningGlobalGain,...
    TargetImpactTime,KinematicMode, RScapPositionSetpointY, RScapStartPositionX,...
    RScapStartPositionY, RScapVCGainX,RScapVCGainY, RScapPCGainX, RScapPCGainY,...
    ZVCFRScapTorqueX, ZVCFRScapTorqueY, ...
    TargetRScapPositionY, TargetRScapVelocityX, TargetRScapVelocityY,...
    RScapAoX, RScapAoY, RScapDampeningX, RScapDampeningY, RScapPositionX,...
    RScapPositionY, RScapVelocityX, RScapVelocityY, RScapStartVelocityX, RScapStartVelocityY,...
    RScapAfX, RScapAfY,RScapInputXD, RScapInputXE, RScapInputXF, RScapInputXG,...
RScapInputYD, RScapInputYE, RScapInputYF, RScapInputYG)

%Tau=Time/TargetImpactTime;
t=Time;

% %%%%%%%%%%%%%%%%%%%%%%%%%%%%%%%%%%%%%%%%%%%
% % Kinetic Input Selection and Calculation
% %%%%%%%%%%%%%%%%%%%%%%%%%%%%%%%%%%%%%%%%%%%

if ModelingMode==0
    % Values are all set to zero.
    JointTorqueRScapX=0;
    JointTorqueRScapY=0;
elseif ModelingMode==1
    % Control based strategy. Values are based on difference in value
    % between the current state and desired state.
    % RScap Joint Rotational Deltas
    DeltaRScapPositionX=RScapPositionX-TargetRScapPositionX;
    DeltaRScapPositionY=RScapPositionY-TargetRScapPositionY;
    DeltaRScapVelocityX=RScapVelocityX-TargetRScapVelocityX;
    DeltaRScapVelocityY=RScapVelocityY-TargetRScapVelocityY;
    % Control Based Strategy
    JointTorqueRScapX=DeltaRScapPositionX*RScapPCGainX*GlobalPCGain-DeltaRScapVelocityX*RScapVCGainX*GlobalVCGain-DampeningGlobalGain*RScapDampeningX*RScapVelocityX;
    JointTorqueRScapY=DeltaRScapPositionY*RScapPCGainY*GlobalPCGain-DeltaRScapVelocityY*RScapVCGainY*GlobalVCGain-DampeningGlobalGain*RScapDampeningY*RScapVelocityY;
elseif ModelingMode==2
    % Forward Dynamics Based Strategy. Values are computed based on a
    % polynomial and a combination of dampening and position gained
    % factors.
    JointTorqueRScapX=Killswitch*GlobalGain*(RScapConstantX+RScapTimeGainX*Time-RScapPositionGainX*(RScapPositionX-RScapPositionSetpointX)...
    -RScapDampeningX*RScapVelocityX);
    JointTorqueRScapY=Killswitch*GlobalGain*(RScapConstantY+RScapTimeGainY*Time-RScapPositionGainY*(RScapPositionY-RScapPositionSetpointY)...
    -RScapDampeningY*RScapVelocityY);
elseif ModelingMode==3
    JointTorqueRScapX=HexPolyInputFunction(RScapInputXA,RScapInputXB,RScapInputXC,RScapInputXD,RScapInputXE,RScapInputXF,RScapInputXG,Time)*Killswitch;
    JointTorqueRScapY=HexPolyInputFunction(RScapInputYA,RScapInputYB,RScapInputYC,RScapInputYD,RScapInputYE,RScapInputYF,RScapInputYG,Time)*Killswitch;  
else
    %ZVCF Based Joint Torques. Values are pulled from model workspace and
    %held constant.
    JointTorqueRScapX=ZVCFRScapTorqueX;
    JointTorqueRScapY=ZVCFRScapTorqueY;
end

% %%%%%%%%%%%%%%%%%%%%%%%%%%%%%%%%%%%%%%%%%%%
% % Kinematic Input Selection and Calculation
% %%%%%%%%%%%%%%%%%%%%%%%%%%%%%%%%%%%%%%%%%%%

if KinematicMode==0
    % All kinematic values set to zero.
    RScapPositionInputX=0;
    RScapPositionInputY=0;
    RScapVelocityInputX=0;
    RScapVelocityInputY=0;
    RScapAccelerationInputX=0;
    RScapAccelerationInputY=0;
elseif KinematicMode==1
    % 1st Order Acceleration, 2nd Order Velocity, 3rd Order Position Solution
    PTX=TargetRScapPositionX;       
    VTX=TargetRScapVelocityX;
    PTY=TargetRScapPositionY;
    VTY=TargetRScapVelocityY;
    % Define Starting Position and Velocity
    PIX=RScapStartPositionX;
    VIX=RScapStartVelocityX;
    PIY=RScapStartPositionY;
    VIY=RScapStartVelocityY;
    AX=3*((VTX+VIX)*TargetImpactTime-2*(PTX-PIX))/TargetImpactTime^3;         % Constant in position equation
    BX=-2*((VTX+2*VIX)*TargetImpactTime-3*(PTX-PIX))/TargetImpactTime^2;         % Constant in position equation
    CX=VIX;         % Starting Velocity at Time Zero
    DX=PIX;         % Starting Position at Time Zero
    AY=3*((VTY+VIY)*TargetImpactTime-2*(PTY-PIY))/TargetImpactTime^3;         % Constant in position equation
    BY=-2*((VTY+2*VIY)*TargetImpactTime-3*(PTY-PIY))/TargetImpactTime^2;         % Constant in position equation
    CY=VIY;         % Starting Velocity at Time Zero
    DY=PIY;         % Starting Position at Time Zero
    % Equation for position as a function of time
    RScapPositionInputX=AX*Time^3/3+BX*Time^2/2+CX*Time+DX;
    RScapPositionInputY=AY*Time^3/3+BY*Time^2/2+CY*Time+DY;
    RScapVelocityInputX=AX*Time^2+BX*Time+CX;
    RScapVelocityInputY=AY*Time^2+BY*Time+CY;
    RScapAccelerationInputX=2*AX*Time+BX;
    RScapAccelerationInputY=2*AY*Time+BY;
elseif KinematicMode==2
    % 2nd Order Acceleration, 3rd Order Velocity, 4th Order Position Solution
    Tt=TargetImpactTime;
    t=Time;
    PoX=RScapStartPositionX;
    PoY=RScapStartPositionY;
    VoX=RScapStartVelocityX;
    VoY=RScapStartVelocityY;
    PfX=TargetRScapPositionX;
    PfY=TargetRScapPositionY;
    VfX=TargetRScapVelocityX;
    VfY=TargetRScapVelocityY;
    AoX=RScapAoX;
    AoY=RScapAoY;
    RScapPositionInputX=PoX + VoX*t + (AoX*t^2)/2 - (t^3*(4*PoX - 4*PfX + Tt*VfX + 3*Tt*VoX + AoX*Tt^2))/Tt^3 + (t^4*(6*PoX - 6*PfX + 2*Tt*VfX + 4*Tt*VoX + AoX*Tt^2))/(2*Tt^4);
    RScapPositionInputY=PoY + VoY*t + (AoY*t^2)/2 - (t^3*(4*PoY - 4*PfY + Tt*VfY + 3*Tt*VoY + AoY*Tt^2))/Tt^3 + (t^4*(6*PoY - 6*PfY + 2*Tt*VfY + 4*Tt*VoY + AoY*Tt^2))/(2*Tt^4);
    RScapVelocityInputX=VoX + AoX*t - (3*t^2*(4*PoX - 4*PfX + Tt*VfX + 3*Tt*VoX + AoX*Tt^2))/Tt^3 + (2*t^3*(6*PoX - 6*PfX + 2*Tt*VfX + 4*Tt*VoX + AoX*Tt^2))/Tt^4;
    RScapVelocityInputY=VoY + AoY*t - (3*t^2*(4*PoY - 4*PfY + Tt*VfY + 3*Tt*VoY + AoY*Tt^2))/Tt^3 + (2*t^3*(6*PoY - 6*PfY + 2*Tt*VfY + 4*Tt*VoY + AoY*Tt^2))/Tt^4;
    RScapAccelerationInputX=AoX + (6*t^2*(6*PoX - 6*PfX + 2*Tt*VfX + 4*Tt*VoX + AoX*Tt^2))/Tt^4 - (6*t*(4*PoX - 4*PfX + Tt*VfX + 3*Tt*VoX + AoX*Tt^2))/Tt^3;
    RScapAccelerationInputY=AoY + (6*t^2*(6*PoY - 6*PfY + 2*Tt*VfY + 4*Tt*VoY + AoY*Tt^2))/Tt^4 - (6*t*(4*PoY - 4*PfY + Tt*VfY + 3*Tt*VoY + AoY*Tt^2))/Tt^3;
else
    % 3rd Order Acceleration, 4th Order Velocity, 5th Order Position Solution
    Tt=TargetImpactTime;
    t=Time;
    PoX=RScapStartPositionX;
    PoY=RScapStartPositionY;
    VoX=RScapStartVelocityX;
    VoY=RScapStartVelocityY;
    PfX=TargetRScapPositionX;
    PfY=TargetRScapPositionY;
    VfX=TargetRScapVelocityX;
    VfY=TargetRScapVelocityY;
    AoX=RScapAoX;
    AoY=RScapAoY;
    AfX=RScapAfX;
    AfY=RScapAfY;
    RScapPositionInputX=PoX+VoX*t+(AoX*t^2)/2-(t^5*(12*PoX-12*PfX+6*Tt*VfX+6*Tt*VoX-AfX*Tt^2+AoX*Tt^2))/(2*Tt^5)-(t^3*(20*PoX-20*PfX+8*Tt*VfX+12*Tt*VoX-AfX*Tt^2+3*AoX*Tt^2))/(2*Tt^3)+(t^4*(30*PoX-30*PfX+14*Tt*VfX+16*Tt*VoX-2*AfX*Tt^2+3*AoX*Tt^2))/(2*Tt^4);
    RScapPositionInputY=PoY+VoY*t+(AoY*t^2)/2-(t^5*(12*PoY-12*PfY+6*Tt*VfY+6*Tt*VoY-AfY*Tt^2+AoY*Tt^2))/(2*Tt^5)-(t^3*(20*PoY-20*PfY+8*Tt*VfY+12*Tt*VoY-AfY*Tt^2+3*AoY*Tt^2))/(2*Tt^3)+(t^4*(30*PoY-30*PfY+14*Tt*VfY+16*Tt*VoY-2*AfY*Tt^2+3*AoY*Tt^2))/(2*Tt^4);  
    RScapVelocityInputX=VoX+AoX*t-(5*t^4*(12*PoX-12*PfX+6*Tt*VfX+6*Tt*VoX-AfX*Tt^2+AoX*Tt^2))/(2*Tt^5)-(3*t^2*(20*PoX-20*PfX+8*Tt*VfX+12*Tt*VoX-AfX*Tt^2+3*AoX*Tt^2))/(2*Tt^3)+(2*t^3*(30*PoX-30*PfX+14*Tt*VfX+16*Tt*VoX-2*AfX*Tt^2+3*AoX*Tt^2))/Tt^4;
    RScapVelocityInputY=VoY+AoY*t-(5*t^4*(12*PoY-12*PfY+6*Tt*VfY+6*Tt*VoY-AfY*Tt^2+AoY*Tt^2))/(2*Tt^5)-(3*t^2*(20*PoY-20*PfY+8*Tt*VfY+12*Tt*VoY-AfY*Tt^2+3*AoY*Tt^2))/(2*Tt^3)+(2*t^3*(30*PoY-30*PfY+14*Tt*VfY+16*Tt*VoY-2*AfY*Tt^2+3*AoY*Tt^2))/Tt^4;
    RScapAccelerationInputX=AoX-(3*t*(20*PoX-20*PfX+8*Tt*VfX+12*Tt*VoX-AfX*Tt^2+3*AoX*Tt^2))/Tt^3-(10*t^3*(12*PoX-12*PfX+6*Tt*VfX+6*Tt*VoX-AfX*Tt^2+AoX*Tt^2))/Tt^5+(6*t^2*(30*PoX-30*PfX+14*Tt*VfX+16*Tt*VoX-2*AfX*Tt^2+3*AoX*Tt^2))/Tt^4;
    RScapAccelerationInputY=AoY-(3*t*(20*PoY-20*PfY+8*Tt*VfY+12*Tt*VoY-AfY*Tt^2+3*AoY*Tt^2))/Tt^3-(10*t^3*(12*PoY-12*PfY+6*Tt*VfY+6*Tt*VoY-AfY*Tt^2+AoY*Tt^2))/Tt^5+(6*t^2*(30*PoY-30*PfY+14*Tt*VfY+16*Tt*VoY-2*AfY*Tt^2+3*AoY*Tt^2))/Tt^4;
end

% Calculate Higher Order Derivatives of the Position Outputs
RScapJerkX=gradient(RScapAccelerationInputX,t);
RScapJerkY=gradient(RScapAccelerationInputY,t);
RScapSnapX=gradient(RScapJerkX,t);
RScapSnapY=gradient(RScapJerkY,t);
RScapCrackleX=gradient(RScapSnapX,t);
RScapCrackleY=gradient(RScapSnapY,t);
RScapPopX=gradient(RScapCrackleX,t);
RScapPopY=gradient(RScapCrackleY,t);

== matlab function GolfSwing3D_KineticallyDriven/Left Hand/LW Unit Vector ==
  data: LWv input; LWSpeed output; LWvx input; LWvy input; LWvz input; LWuvx output; LWuvy output; LWuvz output
function [LWSpeed,LWuvx,LWuvy,LWuvz]  = fcn(LWv,LWvx,LWvy,LWvz)

LWSpeed=norm(LWv);
LWuvx=LWvx/LWSpeed;
LWuvy=LWvy/LWSpeed;
LWuvz=LWvz/LWSpeed;

== matlab function GolfSwing3D_KineticallyDriven/Midpoint/MP Unit Vector ==
  data: MPv input; MidHandSpeed output; MPvx input; MPvy input; MPvz input; MPuvx output; MPuvy output; MPuvz output
function [MidHandSpeed,MPuvx,MPuvy,MPuvz]  = fcn(MPv,MPvx,MPvy,MPvz)

MidHandSpeed=norm(MPv);
MPuvx=MPvx/MidHandSpeed;
MPuvy=MPvy/MidHandSpeed;
MPuvz=MPvz/MidHandSpeed;
